simulink model "Example_2_2ODE"  (Simulink 8.0)
settings: Solver=ode45  StartTime=0.0  StopTime=10.0  RelTol=1e-3
InitFcn:
  | K1=-6; K2=-9;
settings Model: Creator=David  LastModifiedBy=David

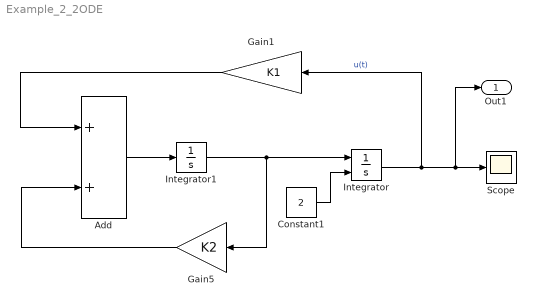
== system Example_2_2ODE ==
  Add : Sum
  Constant1 : Constant  Value=2
  Gain1 : Gain  Gain=K1
  Gain5 : Gain  Gain=K2
  Integrator : Integrator  InitialConditionSource=external  InitialCondition=2
  Integrator1 : Integrator
  Scope : Scope
  Out1 : Outport
  wires:
  Add/1 -> Integrator1/1
  Integrator/1 -> Gain1/1, Out1/1, Scope/1  "u(t)"
  Constant1/1 -> Integrator/2
  Gain1/1 -> Add/1
  Gain5/1 -> Add/2
  Integrator1/1 -> Integrator/1, Gain5/1
